simulink model "Wind_Nordic5_5000MW"  (R2020a)
settings: Solver=ode15s  StartTime=0.0  StopTime=120  MaxStep=1/60  RelTol=1e-2  AbsTol=1e-1  EnableMultiTasking=on
PreLoadFcn:
  | %load_Nordic32_data;
values from neighbouring files (symbols this model uses):
  d_fault = 1400    [load_data_Wind_Nordic5_5000MW_110.m]    (also in load_data_Wind_Nordic5_5000MW_110_sens.m)
  FCR = []    [Wind_fcr_controller_design.m]
  FCR_ideal = []    [Wind_fcr_controller_design.m]
  GenData = table(BUS, type, Td0p,  Td0pp,  Tq0p,   Tq0pp,                     H, Xd, Xq, Xdp, Xqp, Xdpp, Xqpp, XL, Xt,                     BSKV, V0, PGEN, QGEN, QMAX, QMIN, MBASE,                     Ta, vgMAX, gMAX, gMIN, TW, DREF, GenType, GovType)    [load_data_Wind_Nordic5_5000MW_110.m]    (also in load_data_Wind_Nordic5_5000MW_110_sens.m)
  Gwind = []    [load_data_Wind_Nordic5_5000MW_110.m]    (also in load_data_Wind_Nordic5_5000MW_110_sens.m)
  Gwind_speed = []    [load_data_Wind_Nordic5_5000MW_110.m]    (also in load_data_Wind_Nordic5_5000MW_110_sens.m)
  Sgen = Pgen./[0.8;0.8;0.8;0.9;0.9]    [load_data_Wind_Nordic5_5000MW_110.m]    (also in load_data_Wind_Nordic5_5000MW_110_sens.m)
  time_event = time_activate_wind + 5    (= 25)    [load_data_Wind_Nordic5_5000MW_110.m]    (also in load_data_Wind_Nordic5_5000MW_110_sens.m)
  wind_turbines = table(BUS,BSKV,MBASE,POPT,V_WIND,ROT_OPT, ROT_RATED)    [load_data_Wind_Nordic5_5000MW_110.m]    (also in load_data_Wind_Nordic5_5000MW_110_sens.m)
  Wkin = Sgen.*[3;3;3;6;6]    [load_data_Wind_Nordic5_5000MW_110.m]    (also in load_data_Wind_Nordic5_5000MW_110_sens.m)
libraries: Nordic32_Lib x18, powerlib x4
settings Model: Creator=Innocent  LastModifiedBy=joakbj
settings SolverCC: AutoScaleAbsTol=off  MaxOrder=2  ZeroCrossAlgorithm=Adaptive
settings DataIOCC: SaveFormat=Array  SaveOutput=off  SaveTime=off  ReturnWorkspaceOutputs=off
settings OptimizationCC: BlockReduction=off  BooleanDataType=off  ExpressionDepthLimit=2147483647  InitFltsAndDblsToZero=on  LifeSpan=inf
settings DebuggingCC: AlgebraicLoopMsg=none  SaveWithParameterizedLinksMsg=none  UnderspecifiedInitializationDetection=Classic  MergeDetectMultiDrivingBlocksExec=none  SignalResolutionControl=TryResolveAllWithWarning  IgnoredZcDiagnostic=none  MultiTaskDSMMsg=warning  MultiTaskCondExecSysMsg=none  FcnCallInpInsideContextMsg=warning  UnconnectedInputMsg=none  UnconnectedOutputMsg=none  UnconnectedLineMsg=none  StateNameClashWarn=warning  StrictBusMsg=ErrorOnBusTreatedAsVector  SFUnexpectedBacktrackingDiag=warning  SFNoUnconditionalDefaultTransitionDiag=warning  SFExecutionAtInitializationDiag=none  ArithmeticOperatorsInVariantConditions=warning
settings HardwareCC: ProdBitPerPointer=32  ProdBitPerSizeT=32  ProdBitPerPtrDiffT=32  ProdLargestAtomicFloat=None  ProdIntDivRoundTo=Undefined  ProdEndianess=Unspecified  ProdWordSize=32  ProdHWDeviceType=32-bit Generic
settings ModelReferenceCC: PropagateSignalLabelsOutOfModel=off
settings SFSimCC: SimUseLocalCustomCode=off  CustomCodeUndefinedFunction=UseInterfaceOnly
settings RTWCC: RTWUseLocalCustomCode=off
settings CodeAppCC: StateflowObjectComments=on
settings GRTTargetCC: TargetFcnLib=ansi_tfl_tmw.mat  TargetLangStandard=C89/C90 (ANSI)  CombineOutputUpdateFcns=off  GRTInterface=on
settings ConfigComp: CovMetricSettings=dw  CovHtmlReporting=on  CovSaveCumulativeToWorkspaceVar=on  CovSaveSingleToWorkspaceVar=on  CovExternalEMLEnable=off
settings SimscapeCC: SimscapeNormalizeSystem=off

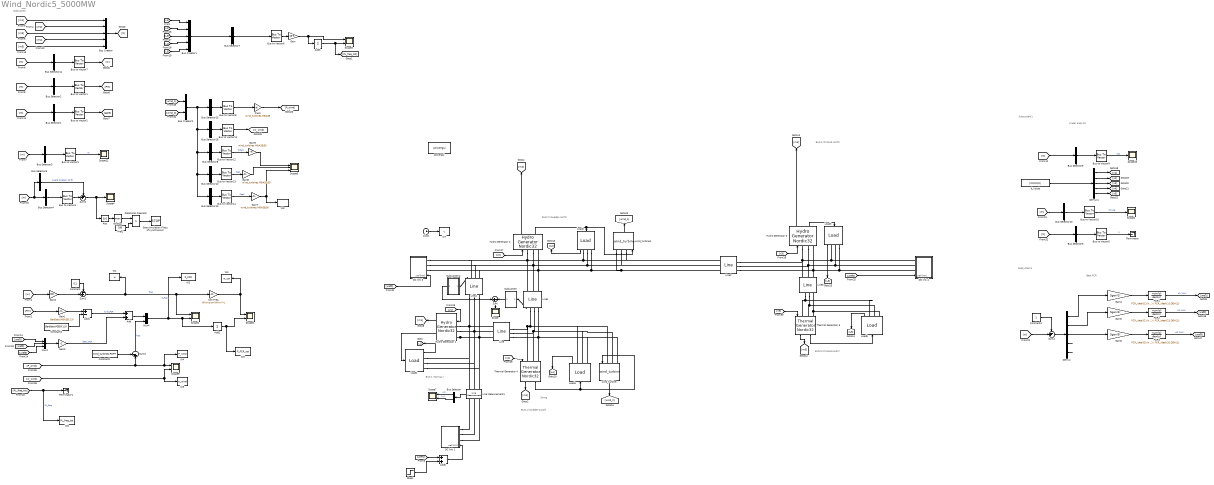
== system Wind_Nordic5_5000MW ==
  note: Subsystem1
  note: Subsystem1
  note: Subsystem
  note: BUS 1 (Norway)
  note: BUS 2 (Sweden-north)
  note: BUS 3 (Finland-north)
  note: BUS 4 (Sweden-south)
  note: BUS 5 (Finland-south)
  note: Swing
  note: Ideal FCR
  note: Linear analysis
  Abs : Abs  SaturateOnIntegerOverflow=on
  Add : Sum
  Add1 : Sum  Inputs=+-
  Add2 : Sum  Inputs=+
  Add3 : Sum  Inputs=+
  Add5 : Sum
  Bus Creator : BusCreator  Inputs=5
  Bus Creator1 : BusCreator  Inputs=5
  Bus Creator2 : BusCreator  Inputs=2
  Bus Selector : BusSelector  OutputSignals=P,V
  Bus Selector1 : BusSelector  OutputSignals=signal1.gate,signal2.gate,signal3.gate  OutputAsBus=on
  Bus Selector10 : BusSelector  OutputSignals=signal1.Pm-Pe,signal2.Pm-Pe,signal3.Pm-Pe,signal4.Pm-Pe,signal5.Pm-Pe  OutputAsBus=on
  Bus Selector11 : BusSelector  OutputSignals="signal1.Rotor speed  wm  (pu),signal2.Rotor speed  wm  (pu),signal3.Rotor speed  wm  (pu),signal4.Rotor speed  wm  (pu),signal5.Rotor speed  wm  (pu)"  OutputAsBus=on
  Bus Selector12 : BusSelector  OutputSignals=signal1.signal6.u,signal2.signal6.u  OutputAsBus=on
  Bus Selector13 : BusSelector  OutputSignals=signal1.signal6.P_set,signal2.signal6.P_set  OutputAsBus=on
  Bus Selector15 : BusSelector  OutputSignals=signal1.Pe/Prated,signal2.Pe/Prated  OutputAsBus=on
  Bus Selector16 : BusSelector  OutputSignals=signal1.w/w_opt,signal2.w/w_opt  OutputAsBus=on
  Bus Selector2 : BusSelector  OutputSignals=signal1.Pm,signal2.Pm,signal3.Pm  OutputAsBus=on
  Bus Selector3 : BusSelector  OutputSignals=signal1.Stator voltage (pu),signal2.Stator voltage (pu),signal3.Stator voltage (pu),signal4.Stator voltage (pu),signal5.Stator voltage (pu)  OutputAsBus=on
  Bus Selector4 : BusSelector  OutputSignals="signal1.Rotor mechanical angle  theta (deg),signal2.Rotor mechanical angle  theta (deg),signal3.Rotor mechanical angle  theta (deg),signal4.Rotor mechanical angle  theta (deg),signal5.Rotor mechanical angle  theta (deg)"  OutputAsBus=on
  Bus Selector5 : BusSelector  OutputSignals="signal1.Rotor mechanical angle  theta (deg)"  OutputAsBus=on
  Bus Selector6 : BusSelector  OutputSignals="signal1.Rotor speed  wm  (pu),signal2.Rotor speed  wm  (pu),signal3.Rotor speed  wm  (pu),signal4.Rotor speed  wm  (pu),signal5.Rotor speed  wm  (pu)"  OutputAsBus=on
  Bus Selector7 : BusSelector  OutputSignals=signal1.PL_freq,signal2.PL_freq,signal3.PL_freq,signal4.PL_freq,signal5.PL_freq  OutputAsBus=on
  Bus Selector8 : BusSelector  OutputSignals=signal1.signal6.P_set_prot,signal2.signal6.P_set_prot  OutputAsBus=on
  Bus Selector9 : BusSelector  OutputSignals=signal1.pss,signal2.pss,signal3.pss,signal4.pss,signal5.pss  OutputAsBus=on
  Bus to Vector{1..14} (14 alike) : BusToVector
  COI Freq : Gain  Gain=Wkin'/sum(Wkin)  Multiplication=Matrix(K*u)
  Clock : Clock
  Constant : Constant  Value=0.1
  Constant1 : Constant  Value=wind_turbines.POPT
  Constant2 : Constant  Value=GenData.PGEN(1:3)
  Constant4 : Constant
  DC link 1 : Subsystem
      settings: PortSchema="{\"entries\":[{\"content\":{\"sides\":[{\"content\":{\"connectorIds\":[\"LConn1\",\"LConn2\",\"LConn3\",\"In1\"]},\"type\":\"ConnectorPlacement.EquallySpacedRectSide\",\"uuid\":\"48445341-a685-4506-9ec8-e376e0c1b939\"},{\"content\":{\"connectorIds\":[],\"side\":\"RIGHT\"},\"type\":\"ConnectorPlacement.EquallySpacedRectSide\",\"uuid\":\"cf3481ef-9523-4ae9-af94-5a03f7da080c\"},{\"content\":{\"connectorIds\":[],\"side\":\"TOP\"},\"type\":\"ConnectorPlacement.EquallySpacedRectSide\",\"uuid\":\"cf4caa18-6df0-400d-a59e-8b335f5a193c\"}]},\"type\":\"ConnectorPlacement.EquallySpacedConnector\",\"uuid\":\"872d10b1-fdd8-4789-878b-9f44ab3824be\"}],\"packageUris\":[\"http://schema.mathworks.com/mf0/Connector/19700101\"],\"version\":\"1.0\"}"
  DC link 3 : Subsystem
      settings: PortSchema="{\"entries\":[{\"content\":{\"sides\":[{\"content\":{\"connectorIds\":[\"LConn1\",\"LConn2\",\"LConn3\",\"In1\"]},\"type\":\"ConnectorPlacement.EquallySpacedRectSide\",\"uuid\":\"48445341-a685-4506-9ec8-e376e0c1b939\"},{\"content\":{\"connectorIds\":[],\"side\":\"RIGHT\"},\"type\":\"ConnectorPlacement.EquallySpacedRectSide\",\"uuid\":\"cf3481ef-9523-4ae9-af94-5a03f7da080c\"},{\"content\":{\"connectorIds\":[],\"side\":\"TOP\"},\"type\":\"ConnectorPlacement.EquallySpacedRectSide\",\"uuid\":\"cf4caa18-6df0-400d-a59e-8b335f5a193c\"}]},\"type\":\"ConnectorPlacement.EquallySpacedConnector\",\"uuid\":\"872d10b1-fdd8-4789-878b-9f44ab3824be\"}],\"packageUris\":[\"http://schema.mathworks.com/mf0/Connector/19700101\"],\"version\":\"1.0\"}"
  DC link 4 : Subsystem
      settings: PortSchema="{\"entries\":[{\"content\":{\"sides\":[{\"content\":{\"connectorIds\":[\"LConn1\",\"LConn2\",\"LConn3\",\"In1\"]},\"type\":\"ConnectorPlacement.EquallySpacedRectSide\",\"uuid\":\"48445341-a685-4506-9ec8-e376e0c1b939\"},{\"content\":{\"connectorIds\":[],\"side\":\"RIGHT\"},\"type\":\"ConnectorPlacement.EquallySpacedRectSide\",\"uuid\":\"cf3481ef-9523-4ae9-af94-5a03f7da080c\"},{\"content\":{\"connectorIds\":[],\"side\":\"TOP\"},\"type\":\"ConnectorPlacement.EquallySpacedRectSide\",\"uuid\":\"cf4caa18-6df0-400d-a59e-8b335f5a193c\"}]},\"type\":\"ConnectorPlacement.EquallySpacedConnector\",\"uuid\":\"872d10b1-fdd8-4789-878b-9f44ab3824be\"}],\"packageUris\":[\"http://schema.mathworks.com/mf0/Connector/19700101\"],\"version\":\"1.0\"}"
  Demux : Demux  Outputs=5
  Demux1 : Demux  Outputs=5
  FCR1 : TransferFcn  Numerator=FCR_ideal{1}.NUM{1}  Denominator=FCR_ideal{1}.DEN{1}
  FCR2 : TransferFcn  Numerator=FCR_ideal{2}.NUM{1}  Denominator=FCR_ideal{2}.DEN{1}
  FCR3 : TransferFcn  Numerator=FCR_ideal{3}.NUM{1}  Denominator=FCR_ideal{3}.DEN{1}
  Gain : Gain  Gain=-1e-6
  Gain1 : Gain  Gain=GenData.MBASE(1:3)
  Gain2 : Gain  Gain=50
  Gain3 : Gain  Gain=-1
  Gain4 : Gain  Gain=Sgen(1)
  Gain5 : Gain  Gain=Sgen(2)
  Gain6 : Gain  Gain=Sgen(3)
  Gain7 : Gain  Gain=wind_turbines.MBASE/50
  Gain8 : Gain  Gain=wind_turbines.MBASE/50
  Gain9 : Gain  Gain=wind_turbines.MBASE/50
  Hydro Generator 1 : Nordic32_Lib/Hydro Generator Nordic32  i=1  gen_data=GenData  pss_data=PSSData  exc_data=ExcData  ii=1  FCR_reg=FCR{1}  fn=fn  open_loop_on=0
      link override Generator: InitialConditions=[0 -39.286 0.805612 0.805612 0.805612 11.7677 -108.232 131.768 1.47939]  BusType=PV
      link override Pref: Value=0.8
      link override Turbine & Regulators/EXCITATION: v0=[1 1.3583]
      link override Turbine & Regulators/Excitation/Excitation Standard: v0=[1 1.4794]
      link override Turbine & Regulators/Hydraulic Turbine and Governor: po=0.8
      link override Turbine & Regulators/Hydraulic Turbine and Governor_modified: po=0.8
      link override Vref: Value=1
  Hydro Generator 2 : Nordic32_Lib/Hydro Generator Nordic32  i=2  gen_data=GenData  pss_data=PSSData  exc_data=ExcData  ii=2  FCR_reg=FCR{2}  fn=fn  open_loop_on=0
      link override Generator: InitialConditions=[0 -11.6088 0.817582 0.817582 0.817582 35.7453 -84.2547 155.745 1.55183]  BusType=PV
      link override Pref: Value=0.8
      link override Turbine & Regulators/EXCITATION: v0=[1 1.3823]
      link override Turbine & Regulators/Excitation/Excitation Standard: v0=[1 1.5518]
      link override Turbine & Regulators/Hydraulic Turbine and Governor: po=0.8
      link override Turbine & Regulators/Hydraulic Turbine and Governor_modified: po=0.8
      link override Vref: Value=1
  Hydro Generator 3 : Nordic32_Lib/Hydro Generator Nordic32  i=3  gen_data=GenData  pss_data=PSSData  exc_data=ExcData  ii=3  FCR_reg=FCR{3}  fn=fn  open_loop_on=0
      link override Generator: InitialConditions=[0 -15.1973 0.80257 0.80257 0.80257 37.4015 -82.5985 157.402 1.44977]  BusType=PV
      link override Pref: Value=0.8
      link override Turbine & Regulators/EXCITATION: v0=[1 1.2705]
      link override Turbine & Regulators/Excitation: K_a=exc_data.K
      link override Turbine & Regulators/Excitation/Excitation Standard: v0=[1 1.4498]
      link override Turbine & Regulators/Hydraulic Turbine and Governor: po=0.8
      link override Turbine & Regulators/Hydraulic Turbine and Governor_modified: po=0.8
      link override Vref: Value=1
  Line : Nordic32_Lib/Line  i=1  data=lines  fn=fn
      link override Distributed Parameters Line: x1=[1.03824651884564e-08 397318.944374014 397319.961593226;314.159265358979 314.159265358979 314.159265358979;2.13511244767427 1.01151737541437 -0.559283140799442]  x2=[6.61585954030749e-08 397657.568884684 397658.451186836;314.159265358979 314.159265358979 314.159265358979;0.0446366991276972 0.665975082184338 -0.904825814894157]  x3=[2.20814826998184e-10 658.401375523783 658.40505590114;314.159265358979 314.159265358979 314.159265358979;-1.38242433795087 -2.27532183546365 2.4370592277969]  x4=[2.18725336325065e-10 3543.58410638642 3543.59485028974;314.159265358979 314.159265358979 314.159265358979;1.40039931788361 0.746410142754541 -0.824391120334144]  x5=0.00124419144739063
  Line Measurement1 : Nordic32_Lib/Line  Measurement  SystemSampleTime=-1  Latency=0  AutoFrameSizeCalculation=off
      settings: PortSchema="{\"entries\":[{\"content\":{\"sides\":[{\"content\":{\"connectorIds\":[\"LConn1\",\"LConn2\",\"LConn3\"]},\"type\":\"ConnectorPlacement.EquallySpacedRectSide\",\"uuid\":\"159cc543-018e-4826-b622-a4d07c97e386\"},{\"content\":{\"connectorIds\":[\"RConn1\",\"RConn2\",\"RConn3\"],\"side\":\"RIGHT\"},\"type\":\"ConnectorPlacement.EquallySpacedRectSide\",\"uuid\":\"cb1aeae8-69bb-45ac-8689-4e8674d58501\"},{\"content\":{\"connectorIds\":[\"Out1\"],\"side\":\"TOP\"},\"type\":\"ConnectorPlacement.EquallySpacedRectSide\",\"uuid\":\"62a962af-3de7-4ff9-a859-7af1186eef9e\"}]},\"type\":\"ConnectorPlacement.EquallySpacedConnector\",\"uuid\":\"81b99b7d-1491-4204-9648-8ec0c780f157\"}],\"packageUris\":[\"http://schema.mathworks.com/mf0/Connector/19700101\"],\"version\":\"1.0\"}"
  Line1 : Nordic32_Lib/Line  i=2  data=lines  fn=fn
      link override Distributed Parameters Line: x1=[2.00716228924775e-08 392930.73841904 392929.79542095;314.159265358979 314.159265358979 314.159265358979;0.298298522450095 1.64832610037767 0.077526318353495]  x2=[6.61585954030749e-08 397657.568884684 397658.451186836;314.159265358979 314.159265358979 314.159265358979;0.257840846988515 0.795997881569382 -0.774803015509113]  x3=[3.42121200488744e-10 9761.00492674746 9761.01940754606;314.159265358979 314.159265358979 314.159265358979;-0.967187256455623 -1.9090565559533 2.8033342935767]  x4=[3.13382468314776e-10 12409.9473851568 12409.9600240636;314.159265358979 314.159265358979 314.159265358979;1.83718087129904 1.21814937621844 -0.352646541650544]  x5=0.000565541566995743
  Line2 : Nordic32_Lib/Line  i=3  data=lines  fn=fn
      link override Distributed Parameters Line: x1=[2.00716228924775e-08 392930.73841904 392929.79542095;314.159265358979 314.159265358979 314.159265358979;0.298298522450095 1.64832610037767 0.077526318353495]  x2=[2.7959609142251e-08 399153.622973644 399152.575688687;314.159265358979 314.159265358979 314.159265358979;0.219242881778632 1.55142327318167 -0.0193744751195984]  x3=[6.72524050180502e-11 315.687122664413 315.697206204013;314.159265358979 314.159265358979 314.159265358979;-0.886162472753078 0.534018505132514 -1.03670017408108]  x4=[6.36421307527972e-11 2761.82970308264 2761.79543104567;314.159265358979 314.159265358979 314.159265358979;1.28155644243314 1.64227693801988 0.0714776211415686]  x5=0.000565541566995743
  Line3 : Nordic32_Lib/Line  i=4  data=lines  fn=fn
      link override Distributed Parameters Line: x1=[2.79688151394615e-08 399153.622973644 399152.575688687;314.159265358979 314.159265358979 314.159265358979;0.12984680769563 1.49724710677124 -0.0735506415300332]  x2=[2.33842089941244e-08 409077.119530648 409076.027281786;314.159265358979 314.159265358979 314.159265358979;0.0482593570782971 1.35974529920149 -0.211050976171259]  x3=[2.41172751708863e-11 370.519428470714 370.526543425891;314.159265358979 314.159265358979 314.159265358979;0.73356611527405 0.494890820170585 -1.0758770821581]  x4=[5.27849699334565e-11 2742.58005284185 2742.55946447589;314.159265358979 314.159265358979 314.159265358979;-0.412171111775138 1.4480361679609 -0.122760709026291]  x5=0.000848312350493614
  Line4 : Nordic32_Lib/Line  i=5  data=lines  fn=fn
      link override Distributed Parameters Line: x1=[1.03824651884564e-08 397318.944374014 397319.961593226;314.159265358979 314.159265358979 314.159265358979;1.9929763491004 0.924835509157671 -0.645965007056138]  x2=[2.00749577753741e-08 392930.73841904 392929.79542095;314.159265358979 314.159265358979 314.159265358979;-0.0567195698831057 1.43162143473593 -0.139178347288245]  x3=[5.12839176441585e-11 3642.76762992647 3642.77086577881;314.159265358979 314.159265358979 314.159265358979;-1.78302732983172 1.05430285699982 -0.51649168271232]  x4=[6.30663702295377e-11 819.737304725572 819.743707033659;314.159265358979 314.159265358979 314.159265358979;1.03528856379174 -1.94646020103311 2.76595127388353]  x5=0.00169662470098723
  Load1 : Nordic32_Lib/Load  i=1  data=loads  fn=fn  local_freq=1
      link override Frequency dependent load: ActiveReactivePowers=[0 0]  PositiveSequence=[1.00835 30.6444]
      link override Three-Phase Dynamic Load: ActiveReactivePowers=[0 0]  PositiveSequence=[0.993298 41.6133]
      link override Three-Phase Parallel C Load: NominalVoltage=(400000)*0.993298
  Load2 : Nordic32_Lib/Load  i=2  data=loads  fn=fn  local_freq=1
      link override Frequency dependent load: ActiveReactivePowers=[0 0]  PositiveSequence=[1 9.84667]
      link override Three-Phase Dynamic Load: ActiveReactivePowers=[0 0]  PositiveSequence=[0.982322 70.6502]
      link override Three-Phase Parallel C Load: NominalVoltage=(400000)*0.982322
  Load3 : Nordic32_Lib/Load  i=3  data=loads  fn=fn  local_freq=1
      link override Frequency dependent load: ActiveReactivePowers=[0 0]  PositiveSequence=[1 9.84667]
      link override Three-Phase Dynamic Load: ActiveReactivePowers=[0 0]  PositiveSequence=[0.997878 65.0982]
      link override Three-Phase Parallel C Load: NominalVoltage=(400000)*0.997878
  Load4 : Nordic32_Lib/Load  i=4  data=loads  fn=fn  local_freq=1
      link override Frequency dependent load: ActiveReactivePowers=[0 0]  PositiveSequence=[1.00485 -12.5262]  NominalVoltage=[ Vn*1e3 fn ]
      link override Three-Phase Dynamic Load: ActiveReactivePowers=[0 0]  PositiveSequence=[0.994143 21.8152]
      link override Three-Phase Parallel C Load: NominalVoltage=(400000)*0.994143
  Load5 : Nordic32_Lib/Load  i=5  data=loads  fn=fn  local_freq=1
      link override Frequency dependent load: ActiveReactivePowers=[0 0]  PositiveSequence=[1.00485 -12.5262]  NominalVoltage=[ Vn*1e3 fn ]
      link override Three-Phase Dynamic Load: ActiveReactivePowers=[0 0]  PositiveSequence=[1.02269 57.2198]
      link override Three-Phase Parallel C Load: NominalVoltage=(400000)*1.02269
  MinMax : MinMax  Function=max  InputSameDT=on  SaturateOnIntegerOverflow=on
  Mux3 : Mux  Inputs=3
  Mux4 : Mux  Inputs=2
  Pnom : Gain  Gain=wind_turbines.MBASE
  Pref2 : Constant  Value=180
  Relational Operator : RelationalOperator  Operator=>  RndMeth=Nearest  InputSameDT=on
  Scope{,2,4,10..11} (5 alike) : Scope
  Scope{1,3,7..9} (5 alike) : Scope  NumInputPorts=2
  Scope5 : Scope  NumInputPorts=3
  Step1 : Step  Time=time_event  After=d_fault  SampleTime=0
  Stop simulation if loss of synchronism : Stop
  Subsystem : Subsystem
  Subsystem2 : Subsystem
  Sum : Sum  Inputs=+-
  Sum{1..4} (4 alike) : Sum  Inputs=-+|
  Terminator : Terminator
  Terminator1 : Terminator
  Thermal Generator 4 : Nordic32_Lib/Thermal Generator Nordic32  i=4  gen_data=GenData  pss_data=PSSData  exc_data=ExcData  fn=fn
      link override Generator: InitialConditions=[0 -31.2449 0.951758 0.951758 0.951758 -6.54848 -126.548 113.452 2.55075]  BusType=swing
      link override Pref: Value=0.94555
      link override Turbine & Regulators/EXCITATION: v0=[1 2.3668]
      link override Turbine & Regulators/Excitation/Excitation Standard: v0=[1 2.5508]
      link override Vref: Value=1
  Thermal Generator 5 : Nordic32_Lib/Thermal Generator Nordic32  i=5  gen_data=GenData  pss_data=PSSData  exc_data=ExcData  fn=fn
      link override Generator: InitialConditions=[0 12.1541 0.904474 0.904474 0.904474 40.4895 -79.5105 160.49 2.25569]  BusType=PV
      link override Pref: Value=0.9
      link override Turbine & Regulators/EXCITATION: v0=[1 2.3447]
      link override Turbine & Regulators/Excitation/Excitation Standard: v0=[1 2.2557]
      link override Vref: Value=1
  W1 : ToWorkspace  VariableName=w  SampleTime=1/60
  W2 : ToWorkspace  VariableName=P_FCR  SampleTime=1/60
  W3 : ToWorkspace  VariableName=w_coi  SampleTime=1/60
  W4 : ToWorkspace  VariableName=P_wind  SampleTime=1/60
  W5 : ToWorkspace  VariableName=w_wind  SampleTime=1/60
  W6 : ToWorkspace  VariableName=P_FCR_tot  SampleTime=1/60
  W7 : ToWorkspace  VariableName=t  SampleTime=1/60
  W8 : ToWorkspace  VariableName=PL_freq_tot  SampleTime=1/60
  W9 : ToWorkspace  VariableName=P_wind_set  SampleTime=1/60
  d_Vstab : Constant  Value=[0;0;0;0;0]
  powergui : powerlib/powergui  Priority=2  SimulationMode=Phasor  SampleTime=0  frequency=50  Iterations=100  frequencyindice=50  Pbase=100e6  ErrMax=1e-06  UnitsV=kV  UnitsW=MW  buscounter=3  FunctionMessages=off  echomessages=off  EnableUseOfTLC=off  CurrentSourceSwitches=off  DisableSnubberDevices=off  DisableRonSwitches=off  DisableVfSwitches=off  DisplayEquations=off  AutomaticDiscreteSolvers=off  SolverType=Tustin/Backward Euler (TBE)  Interpol=off  ExternalGateDelay=off  methode=off  Ts=100  x0status=blocks  SPID=off  SwTol=0  HookPort=off  NonlinearTolerance=1e-4  nMaxIteration=100  ContinueOnMaxIteration=off  RestoreLinks=warning  ResistiveCurrentMeasurement=off  Frange=logspace(0,3,50)  Ylog=off  Xlog=off  ShowGrid=off  save=off  variable=ZData  structure=0  ZoomFFT=on  StartTime=0.0  cycles=1  DisplayStyle=1  fundamental=60  FreqAxis=off  MaxFrequency=1000  frequencyindicesteady=1  RmsSteady=1  display=off
  wind_turbine : Nordic32_Lib/wind_turbine  i=2  data=wind_turbines  data_NREL=data_NREL  fn=fn  time_activate_wind=time_activate_wind  Gwind=Gwind{2}  Gwind_speed=Gwind_speed{2}  FCR=FCR{5}
      link override Three-Phase Dynamic Load2: ActiveReactivePowers=[0 0]  PositiveSequence=[0.994143 21.8152]
  wind_turbine1 : Nordic32_Lib/wind_turbine  i=1  data=wind_turbines  data_NREL=data_NREL  fn=fn  time_activate_wind=time_activate_wind  Gwind=Gwind{1}  Gwind_speed=Gwind_speed{1}  FCR=FCR{4}
      link override Three-Phase Dynamic Load2: ActiveReactivePowers=[0 0]  PositiveSequence=[0.982322 70.6502]
  wires:
  Clock/1 -> W7/1
  Thermal Generator 4/1 -> [m4]
  Thermal Generator 4/2 -> wind_turbine/1, Load4/1
  [Pm] -> Gain1/1
  [w] -> Gain2/1
  Hydro Generator 1/2 -> Load1/1
  Hydro Generator 1/1 -> [m1]
  Hydro Generator 2/2 -> wind_turbine1/1, Load2/1
  Hydro Generator 2/1 -> [m2]
  Hydro Generator 3/1 -> [m3]
  Hydro Generator 3/2 -> Load3/1
  Thermal Generator 5/2 -> Load5/1
  Thermal Generator 5/1 -> [m5]
  Gain2/1 -> Sum1/2
  Sum1/1 -> W1/1, Scope1/1, COI Freq/1  "freq"
  Constant/1 -> Sum1/1
  Gain1/1 -> Add1/1
  Constant2/1 -> Add1/2
  Load1/1 -> [L1]
  Load4/1 -> [L4]
  Load5/1 -> [L5]
  Load3/1 -> [L3]
  [L1] -> Bus Creator1/1
  [L2] -> Bus Creator1/2
  [L3] -> Bus Creator1/3
  [L4] -> Bus Creator1/4
  [L5] -> Bus Creator1/5
  Bus Creator1/1 -> Bus Selector7/1
  [uref1] -> Mux3/1
  [uref2] -> Mux3/2
  [uref3] -> Mux3/3
  Mux3/1 -> Gain3/1
  [uref1] -> Add5/1
  [m3] -> Bus Creator/3
  Bus Selector4/1 -> Bus to Vector4/1
  Bus Selector5/1 -> Sum2/1  "Angle Sweden North"
  Bus to Vector1/1 -> [Pm]
  [m] -> Bus Selector2/1
  [m5] -> Bus Creator/5
  [m4] -> Bus Creator/4
  [m1] -> Bus Creator/1
  Bus Selector3/1 -> Bus to Vector3/1
  Bus to Vector4/1 -> Sum2/2
  Bus to Vector3/1 -> Scope11/1  "Vt"
  [m] -> Bus Selector5/1, Bus Selector4/1
  Bus Creator/1 -> [m]
  Bus to Vector2/1 -> [gate]
  [m] -> Bus Selector11/1
  Bus Selector1/1 -> Bus to Vector2/1
  [m] -> Bus Selector3/1
  [m2] -> Bus Creator/2
  Bus Selector11/1 -> Bus to Vector7/1
  Sum2/1 -> Abs/1, Scope4/1
  [m] -> Bus Selector1/1
  Bus Selector2/1 -> Bus to Vector1/1
  Bus to Vector7/1 -> [w]
  Line1/1 -> Subsystem/1(In1)
  Subsystem/1(Out1) -> Sum/2
  Add5/1 -> DC link 1/1(uref [MW])
  Step1/1 -> Add5/2
  [uref2] -> DC link 3/1(uref [MW])
  [uref3] -> DC link 4/1(uref [MW])
  Bus to Vector6/1 -> Gain/1
  Bus Selector7/1 -> Bus to Vector6/1
  Add3/1 -> [PL_freq_tot], Scope3/2
  [v1] -> Hydro Generator 1/2
  [v2] -> Hydro Generator 2/2
  [v3] -> Hydro Generator 3/2
  [v4] -> Thermal Generator 4/1
  [v5] -> Thermal Generator 5/1
  Line Measurement1/1 -> Bus Selector/1
  Bus Selector/1 -> Scope7/1  "<P>"
  Bus Selector/2 -> Scope7/2  "<V>"
  [PL_freq_tot] -> W8/1, Terminator1/1  "PL_freq"
  Gain/1 -> Add3/1, Scope3/1
  Line4/1 -> Subsystem2/1(In1)
  Subsystem2/1(Out1) -> Sum/1
  Sum/1 -> Scope/1
  FCR2/1 -> [uref2]  "d2 (MW)"
  Demux/1 -> Gain4/1
  Demux/5 -> ?
  [w] -> Sum4/2
  Demux/2 -> Gain5/1
  Constant4/1 -> Sum4/1
  Gain5/1 -> FCR2/1
  FCR3/1 -> [uref3]  "d3 (MW)"
  FCR1/1 -> [uref1]  "d1 (MW)"
  Sum4/1 -> Demux/1
  Demux/3 -> Gain6/1
  Gain6/1 -> FCR3/1
  Demux/4 -> ?
  Gain4/1 -> FCR1/1
  Demux1/1 -> [v1]
  Bus Selector9/1 -> Bus to Vector9/1
  d_Vstab/1 -> Demux1/1
  Bus to Vector5/1 -> Terminator/1  "w"
  Demux1/3 -> [v3]
  [m] -> Bus Selector6/1
  [m] -> Bus Selector9/1
  Bus to Vector10/1 -> Scope2/1  "Pm-Pe"
  Demux1/4 -> [v4]
  Bus Selector6/1 -> Bus to Vector5/1
  Demux1/2 -> [v2]
  [m] -> Bus Selector10/1
  Bus to Vector9/1 -> Scope10/1  "pss"
  Bus Selector10/1 -> Bus to Vector10/1
  Demux1/5 -> [v5]
  Load2/1 -> [L2]
  Abs/1 -> MinMax/1
  Pref2/1 -> Relational Operator/2
  Relational Operator/1 -> Stop simulation if loss of synchronism/1
  MinMax/1 -> Relational Operator/1
  wind_turbine1/2 -> [wind_1]
  wind_turbine/2 -> [wind_2]
  Add1/1 -> Add/1  "hydr_FCR"
  Gain3/1 -> Add/2  "ideal_FCR"
  Mux4/1 -> Add2/1, Scope1/2, W2/1  "P_FCR"
  COI Freq/1 -> Scope8/1, W3/1
  [wind_1] -> Bus Creator2/1
  [wind_2] -> Bus Creator2/2
  Bus Creator2/1 -> Bus Selector13/1, Bus Selector12/1, Bus Selector8/1, Bus Selector16/1, Bus Selector15/1
  Bus Selector15/1 -> Bus to Vector8/1
  Bus to Vector8/1 -> Pnom/1
  Bus Selector16/1 -> Bus to Vector11/1
  Pnom/1 -> [P_wind]
  Bus to Vector11/1 -> [w_wind]
  Add/1 -> Mux4/1
  [P_wind] -> Sum3/2, W4/1, Scope9/1
  Add2/1 -> W6/1, Scope8/2
  [w_wind] -> Scope9/2, W5/1
  Sum3/1 -> Mux4/2  "freq"
  Constant1/1 -> Sum3/1
  Bus Selector8/1 -> Bus to Vector12/1
  Bus Selector12/1 -> Bus to Vector13/1
  Bus Selector13/1 -> Bus to Vector14/1
  Bus to Vector13/1 -> Gain8/1  "Pset"
  Bus to Vector12/1 -> Gain9/1  "Pstab"
  Bus to Vector14/1 -> Gain7/1  "Pset'"
  Gain7/1 -> W9/1, Scope5/3
  Gain8/1 -> Scope5/2
  Gain9/1 -> Scope5/1
  connections:
  Thermal Generator 4/LConn3 -- wind_turbine/LConn3 -- Load4/RConn3 -- Line1/RConn3 -- Line/RConn3
  Thermal Generator 4/LConn2 -- wind_turbine/LConn2 -- Load4/RConn2 -- Line1/RConn2 -- Line/RConn2
  Line1/RConn1 -- wind_turbine/LConn1 -- Load4/RConn1 -- Thermal Generator 4/LConn1 -- Line/RConn1
  Hydro Generator 1/LConn3 -- Line Measurement1/RConn3 -- Load1/RConn3 -- Line/LConn3 -- Line4/LConn3
  Hydro Generator 1/LConn2 -- Line Measurement1/RConn2 -- Load1/RConn2 -- Line/LConn2 -- Line4/LConn2
  Hydro Generator 2/LConn1 -- wind_turbine1/LConn1 -- Line2/LConn1 -- Load2/RConn1 -- DC link 3/LConn1 -- Line4/RConn1 -- Line1/LConn1
  Line2/LConn3 -- wind_turbine1/LConn3 -- Load2/RConn3 -- Hydro Generator 2/LConn3 -- Line1/LConn3 -- DC link 3/LConn3 -- Line4/RConn3
  Hydro Generator 2/LConn2 -- wind_turbine1/LConn2 -- Line2/LConn2 -- Load2/RConn2 -- Line1/LConn2 -- DC link 3/LConn2 -- Line4/RConn2
  Hydro Generator 3/LConn2 -- Line2/RConn2 -- Line3/LConn2 -- DC link 4/LConn2 -- Load3/RConn2
  Load3/RConn3 -- Hydro Generator 3/LConn3 -- Line2/RConn3 -- Line3/LConn3 -- DC link 4/LConn3
  Hydro Generator 3/LConn1 -- Line2/RConn1 -- Line3/LConn1 -- DC link 4/LConn1 -- Load3/RConn1
  Thermal Generator 5/LConn3 -- Load5/RConn3 -- Line3/RConn3
  Line3/RConn2 -- Load5/RConn2 -- Thermal Generator 5/LConn2
  Line3/RConn1 -- Load5/RConn1 -- Thermal Generator 5/LConn1
  Line/LConn1 -- Line Measurement1/RConn1 -- Load1/RConn1 -- Hydro Generator 1/LConn1 -- Line4/LConn1
  DC link 1/LConn1 -- Line Measurement1/LConn1
  DC link 1/LConn2 -- Line Measurement1/LConn2
  DC link 1/LConn3 -- Line Measurement1/LConn3

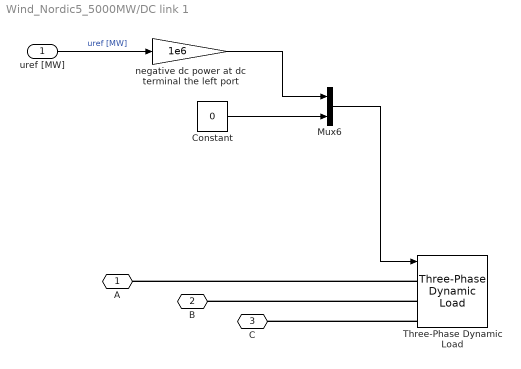
== system Wind_Nordic5_5000MW/DC link 1 ==
  uref [MW] : Inport
  Constant : Constant  Value=0
  Mux6 : Mux  Inputs=2
  Three-Phase Dynamic Load : powerlib/Elements/Three-Phase Dynamic Load  NominalVoltage=[ 400e3 50 ]  ActiveReactivePowers=[0 0]  PositiveSequence=[0.993298 41.6133]  ExternalControl=on  NpNq=[1.3 2]  TimeConstants="[0  0  0  0]"  MinimumVoltage=0.7  Tfilter=1e-4  LoadFlowParameters=[4,0,0,0,0]
      settings: SourceProductBaseCode=PS
  negative dc power at dc terminal the left port : Gain  Gain=1e6
  A : PMIOPort  Side=Left
  B : PMIOPort  Port=2  Side=Left
  C : PMIOPort  Port=3  Side=Left
  wires:
  Constant/1 -> Mux6/2
  Mux6/1 -> Three-Phase Dynamic Load/1
  negative dc power at dc terminal the left port/1 -> Mux6/1
  uref [MW]/1 -> negative dc power at dc terminal the left port/1  "uref [MW]"
  connections:
  Three-Phase Dynamic Load/LConn1 -- A/RConn1
  Three-Phase Dynamic Load/LConn2 -- B/RConn1
  Three-Phase Dynamic Load/LConn3 -- C/RConn1

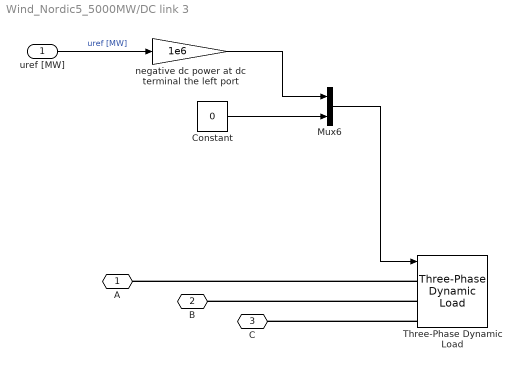
== system Wind_Nordic5_5000MW/DC link 3 ==
  uref [MW] : Inport
  Constant : Constant  Value=0
  Mux6 : Mux  Inputs=2
  Three-Phase Dynamic Load : powerlib/Elements/Three-Phase Dynamic Load  NominalVoltage=[ 400e3 50 ]  ActiveReactivePowers=[0 0]  PositiveSequence=[0.982322 70.6502]  ExternalControl=on  NpNq=[1.3 2]  TimeConstants="[0  0  0  0]"  MinimumVoltage=0.7  Tfilter=1e-4  LoadFlowParameters=[4,0,0,0,0]
      settings: SourceProductBaseCode=PS
  negative dc power at dc terminal the left port : Gain  Gain=1e6
  A : PMIOPort  Side=Left
  B : PMIOPort  Port=2  Side=Left
  C : PMIOPort  Port=3  Side=Left
  wires:
  Constant/1 -> Mux6/2
  Mux6/1 -> Three-Phase Dynamic Load/1
  negative dc power at dc terminal the left port/1 -> Mux6/1
  uref [MW]/1 -> negative dc power at dc terminal the left port/1  "uref [MW]"
  connections:
  Three-Phase Dynamic Load/LConn1 -- A/RConn1
  Three-Phase Dynamic Load/LConn2 -- B/RConn1
  Three-Phase Dynamic Load/LConn3 -- C/RConn1

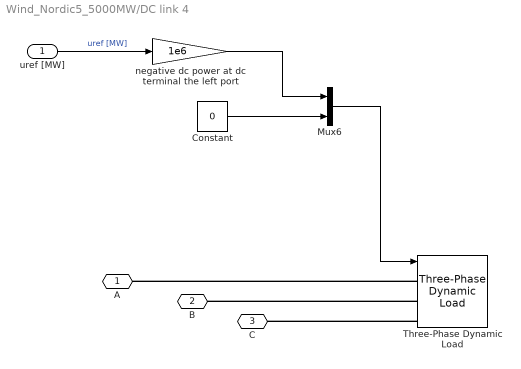
== system Wind_Nordic5_5000MW/DC link 4 ==
  uref [MW] : Inport
  Constant : Constant  Value=0
  Mux6 : Mux  Inputs=2
  Three-Phase Dynamic Load : powerlib/Elements/Three-Phase Dynamic Load  NominalVoltage=[ 400e3 50 ]  ActiveReactivePowers=[0 0]  PositiveSequence=[0.997878 65.0982]  ExternalControl=on  NpNq=[1.3 2]  TimeConstants="[0  0  0  0]"  MinimumVoltage=0.7  Tfilter=1e-4  LoadFlowParameters=[4,0,0,0,0]
      settings: SourceProductBaseCode=PS
  negative dc power at dc terminal the left port : Gain  Gain=1e6
  A : PMIOPort  Side=Left
  B : PMIOPort  Port=2  Side=Left
  C : PMIOPort  Port=3  Side=Left
  wires:
  Constant/1 -> Mux6/2
  Mux6/1 -> Three-Phase Dynamic Load/1
  negative dc power at dc terminal the left port/1 -> Mux6/1
  uref [MW]/1 -> negative dc power at dc terminal the left port/1  "uref [MW]"
  connections:
  Three-Phase Dynamic Load/LConn1 -- A/RConn1
  Three-Phase Dynamic Load/LConn2 -- B/RConn1
  Three-Phase Dynamic Load/LConn3 -- C/RConn1

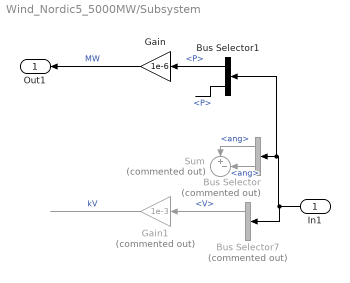
== system Wind_Nordic5_5000MW/Subsystem ==
  In1 : Inport
  Bus Selector : BusSelector  Commented=on  OutputSignals=signal1.ang,signal2.ang
  Bus Selector1 : BusSelector  OutputSignals=signal1.P,signal2.P
  Bus Selector7 : BusSelector  Commented=on  OutputSignals=signal1.V,signal2.V
  Gain : Gain  Gain=1e-6
  Gain1 : Gain  Commented=on  Gain=1e-3
  Sum : Sum  Commented=on  Inputs=+-|
  Out1 : Outport
  wires:
  In1/1 -> Bus Selector7/1, Bus Selector1/1, Bus Selector/1
  Bus Selector7/1 -> Gain1/1  "<V>"
  Bus Selector/2 -> Sum/2  "<ang>"
  Bus Selector/1 -> Sum/1  "<ang>"
  Bus Selector1/1 -> Gain/1  "<P>"
  Bus Selector1/2 -> ?  "<P>"
  Gain/1 -> Out1/1  "MW"
  Gain1/1 -> ?  "kV"

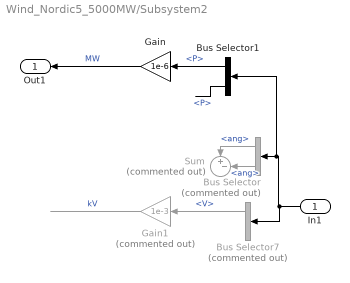
== system Wind_Nordic5_5000MW/Subsystem2 ==
  In1 : Inport
  Bus Selector : BusSelector  Commented=on  OutputSignals=signal1.ang,signal2.ang
  Bus Selector1 : BusSelector  OutputSignals=signal1.P,signal2.P
  Bus Selector7 : BusSelector  Commented=on  OutputSignals=signal1.V,signal2.V
  Gain : Gain  Gain=1e-6
  Gain1 : Gain  Commented=on  Gain=1e-3
  Sum : Sum  Commented=on  Inputs=+-|
  Out1 : Outport
  wires:
  In1/1 -> Bus Selector7/1, Bus Selector1/1, Bus Selector/1
  Bus Selector7/1 -> Gain1/1  "<V>"
  Bus Selector/2 -> Sum/2  "<ang>"
  Bus Selector/1 -> Sum/1  "<ang>"
  Bus Selector1/1 -> Gain/1  "<P>"
  Bus Selector1/2 -> ?  "<P>"
  Gain/1 -> Out1/1  "MW"
  Gain1/1 -> ?  "kV"
